simulink model "q2simulink"  (R2023b)
settings: Solver=VariableStepAuto  StartTime=0.0  StopTime=35  RelTol=1e-3
values from neighbouring files (symbols this model uses):
  den1 = conv(den1, [La+Lf Ra+Rf])    [q2file.m]
  den2 = conv(den2, [La+Lf Ra+Rf])    [q2file.m]
  den_i = [(La+Lf) (Ra+Rf)]    [q2file.m]
  den_v = [J B]    [q2file.m]
  dk2 = [T2 1]    [q2file.m]
  K1 = abs(1/(k1*gp1))    [q2file.m]
  Ka = 0.2    [q2file.m]
  Kc = 4    [q2file.m]
  nk2 = [alfa2*T2 1]    [q2file.m]
  num1 = Ka    (= 0.2)    [q2file.m]
  num2 = Ka    (= 0.2)    [q2file.m]
  num_i = 1    [q2file.m]
  num_v = 1    [q2file.m]
  p_c1 = Re_s1-(Im_s1/tan((pi/180)*theta_p1))    [q2file.m]
  z_c1 = Re_s1-(Im_s1/tan((pi/180)*theta_z1))    [q2file.m]
settings Model: Creator=klysm  LastModifiedBy=klysm

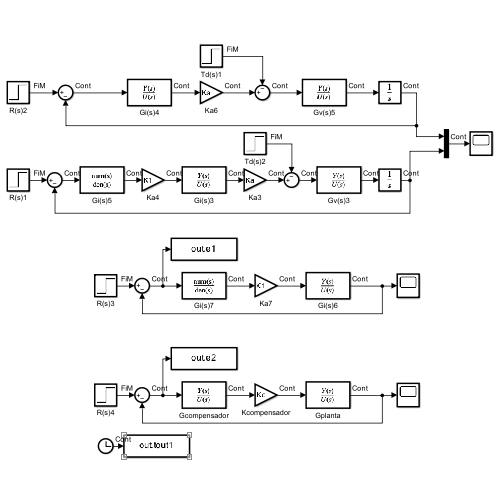
[thumbnail: Simulink's stored preview of the top-level diagram]
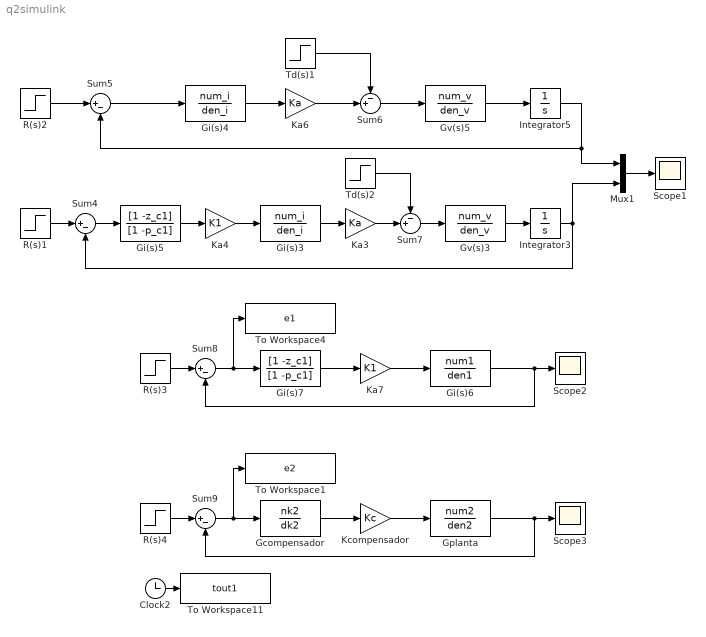
== system q2simulink ==
  Clock2 : Clock
      settings: Decimation=20
  Gcompensador : TransferFcn  Numerator=nk2  Denominator=dk2
  Gi(s)3 : TransferFcn  Numerator=num_i  Denominator=den_i
  Gi(s)4 : TransferFcn  Numerator=num_i  Denominator=den_i
  Gi(s)5 : TransferFcn  Numerator=[1 -z_c1]  Denominator=[1 -p_c1]
  Gi(s)6 : TransferFcn  Numerator=num1  Denominator=den1
  Gi(s)7 : TransferFcn  Numerator=[1 -z_c1]  Denominator=[1 -p_c1]
  Gplanta : TransferFcn  Numerator=num2  Denominator=den2
  Gv(s)3 : TransferFcn  Numerator=num_v  Denominator=den_v
  Gv(s)5 : TransferFcn  Numerator=num_v  Denominator=den_v
  Integrator3 : Integrator
  Integrator5 : Integrator
  Ka3 : Gain  Gain=Ka
  Ka4 : Gain  Gain=K1
  Ka6 : Gain  Gain=Ka
  Ka7 : Gain  Gain=K1
  Kcompensador : Gain  Gain=Kc
  Mux1 : Mux  Inputs=2
  R(s){1..4} (4 alike) : Step  SampleTime=0
  Scope1 : Scope
  Scope2 : Scope
  Scope3 : Scope
  Sum{4..5,8..9} (4 alike) : Sum  Inputs=|+-
  Sum6 : Sum  Inputs=-+|
  Sum7 : Sum  Inputs=-+|
  Td(s)1 : Step  SampleTime=0
  Td(s)2 : Step  SampleTime=0
  To Workspace1 : ToWorkspace  VariableName=e2  SampleTime=-1
  To Workspace11 : ToWorkspace  VariableName=tout1  SampleTime=-1
  To Workspace4 : ToWorkspace  VariableName=e1  SampleTime=-1
  wires:
  Integrator3/1 -> Sum4/2, Mux1/2
  R(s)1/1 -> Sum4/1
  R(s)2/1 -> Sum5/1
  Integrator5/1 -> Mux1/1, Sum5/2
  Mux1/1 -> Scope1/1
  Td(s)1/1 -> Sum6/1
  Gv(s)5/1 -> Integrator5/1
  Ka6/1 -> Sum6/2
  Gi(s)4/1 -> Ka6/1
  Sum6/1 -> Gv(s)5/1
  Sum5/1 -> Gi(s)4/1
  Gi(s)5/1 -> Ka4/1
  Gv(s)3/1 -> Integrator3/1
  Gi(s)3/1 -> Ka3/1
  Td(s)2/1 -> Sum7/1
  Sum7/1 -> Gv(s)3/1
  Ka3/1 -> Sum7/2
  Sum4/1 -> Gi(s)5/1
  Ka4/1 -> Gi(s)3/1
  Ka7/1 -> Gi(s)6/1
  R(s)3/1 -> Sum8/1
  Gi(s)7/1 -> Ka7/1
  Gi(s)6/1 -> Scope2/1, Sum8/2
  Gplanta/1 -> Scope3/1, Sum9/2
  Gcompensador/1 -> Kcompensador/1
  Kcompensador/1 -> Gplanta/1
  R(s)4/1 -> Sum9/1
  Clock2/1 -> To Workspace11/1
  Sum8/1 -> To Workspace4/1, Gi(s)7/1
  Sum9/1 -> To Workspace1/1, Gcompensador/1
